simulink model "Gravity_model"  (R2025b)
settings: Solver=FixedStepDiscrete  StartTime=0.0  StopTime=50  FixedStep=0.01  RelTol=1e-3
undefined symbols (not defined in the file): Earth_mu, Earth_radius
settings Model: DataDictionary=Environment_data.sldd  Creator=mauro  LastModifiedBy=mauro
settings DataIOCC: SaveOutput=off  SaveTime=off

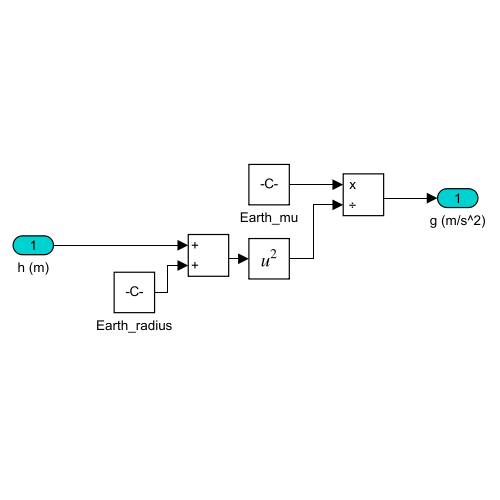
[thumbnail: Simulink's stored preview of the top-level diagram]
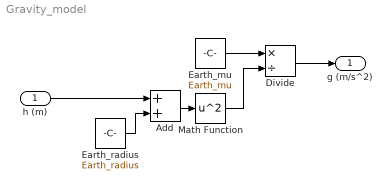
== system Gravity_model ==
  h (m) : Inport  OutDataTypeStr=double  PortDimensions=1
  Add : Sum
  Divide : Product  Inputs=*/
  Earth_mu : Constant  Value=Earth_mu
  Earth_radius : Constant  Value=Earth_radius
  Math Function : Math  Operator=square
  g (m/s^2) : Outport  OutDataTypeStr=double  PortDimensions=1
  wires:
  Earth_radius/1 -> Add/2
  Add/1 -> Math Function/1
  Earth_mu/1 -> Divide/1
  Math Function/1 -> Divide/2
  h (m)/1 -> Add/1
  Divide/1 -> g (m/s^2)/1
